simulink model "LED_Blinker_NoPulse"  (R2025a)
settings: Solver=VariableStepAuto  StartTime=0.0  StopTime=10.0  RelTol=1e-3
libraries: simulink x1
settings Model: Creator=mahij  LastModifiedBy=mahij

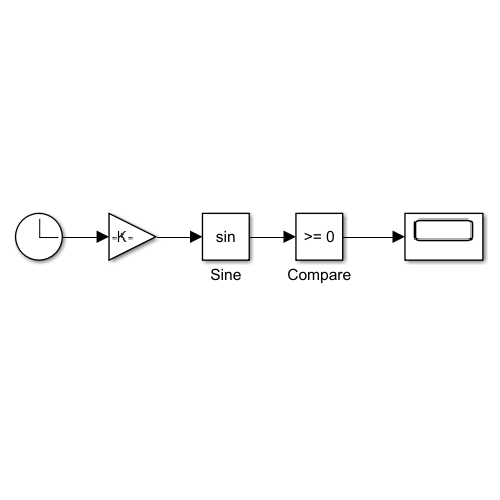
[thumbnail: Simulink's stored preview of the top-level diagram]
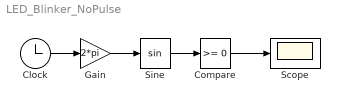
== system LED_Blinker_NoPulse ==
  Clock : Clock
  Compare : simulink/Logic and Bit Operations/Compare To Constant  relop=>=  const=0  OutDataTypeStr=boolean
  Gain : Gain  Gain=2*pi
  Scope : Scope
  Sine : Trigonometry
  wires:
  Clock/1 -> Gain/1
  Gain/1 -> Sine/1
  Sine/1 -> Compare/1
  Compare/1 -> Scope/1
